simulink subsystem "quantile_effort_controller"  (R2024b)
settings: Solver=VariableStepAuto  StartTime=0.0  StopTime=10.0  RelTol=1e-3
undefined symbols (not defined in the file): const_brake, controller_rate
settings Model: Creator=yevge  LastModifiedBy=Aiden Gaydos

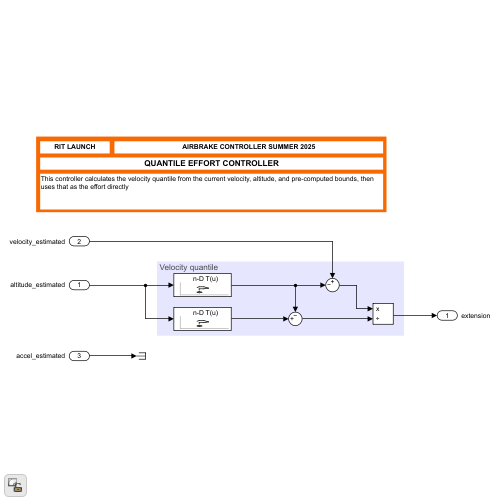
[thumbnail: Simulink's stored preview of the top-level diagram]
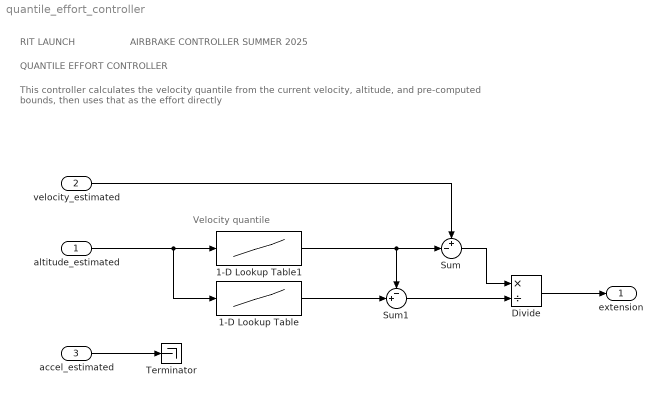
== system quantile_effort_controller ==
  note: Velocity quantile
  note: QUANTILE EFFORT CONTROLLER
  note: This controller calculates the velocity quantile from the current velocity, altitude, and pre-computed bounds, then uses that as the effort directly
  note: RIT LAUNCH
  note: AIRBRAKE CONTROLLER SUMMER 2025
  altitude_estimated : Inport  Unit=m  PortDimensions=1
  velocity_estimated : Inport  Port=2  Unit=m/s  PortDimensions=1
  accel_estimated : Inport  Port=3  Unit=m/s^2  PortDimensions=1
  1-D Lookup Table : Lookup_n-D  NumberOfTableDimensions=1  DataSpecification=Lookup table object  LookupTableObject=upper_bound_lut  BreakpointsForDimension1=[-5:5]  Table=tanh([-5:5])  InternalRulePriority=Speed  RndMeth=Simplest
  1-D Lookup Table1 : Lookup_n-D  NumberOfTableDimensions=1  DataSpecification=Lookup table object  LookupTableObject=lower_bound_lut  BreakpointsForDimension1=[-5:5]  Table=tanh([-5:5])  InternalRulePriority=Speed  RndMeth=Simplest
  Divide : Product  Inputs=*/
  Sum : Sum  Inputs=+-|
  Sum1 : Sum  Inputs=-+|
  Terminator : Terminator
  extension : Outport  Unit=1  PortDimensions=1  SampleTime=1/controller_rate  InitialOutput=const_brake
  wires:
  accel_estimated/1 -> Terminator/1
  Divide/1 -> extension/1
  altitude_estimated/1 -> 1-D Lookup Table/1, 1-D Lookup Table1/1
  1-D Lookup Table1/1 -> Sum1/1, Sum/2
  1-D Lookup Table/1 -> Sum1/2
  Sum/1 -> Divide/1
  Sum1/1 -> Divide/2
  velocity_estimated/1 -> Sum/1
